simulink model "project3_v1_CoSim"  (R2021a)
settings: Solver=VariableStepAuto  StartTime=0.0  StopTime=30  RelTol=1e-3
undefined symbols (not defined in the file or in its folder): A, N
libraries: hdlBasic x25, xbsIndex_r4 x1, JTAGRuntimeCosim_r4 x1
settings Model: Creator=caval  LastModifiedBy=hl116

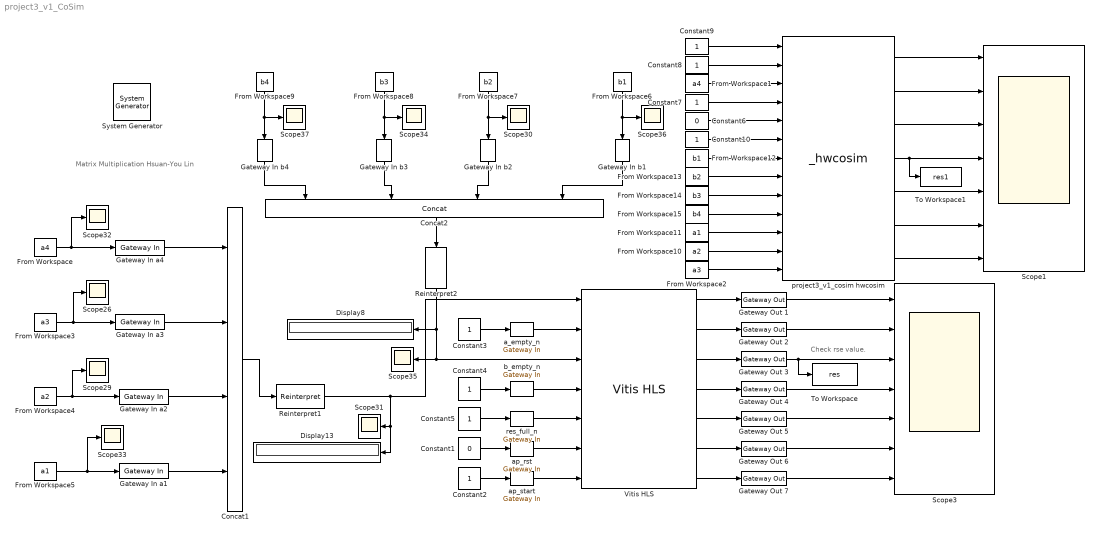
== system project3_v1_CoSim ==
  note: Matrix Multiplication
      | Hsuan-You Lin
  note: Check rse value.
  " System Generator" : xbsIndex_r4/ System Generator  Tag=genX  xilinxfamily=zynq  part=xc7z020  speed=-1  package=clg484  synthesis_tool=Vivado  clock_wrapper=Clock Enables  directory=./netlist_cosim  proj_type=Vivado  Synth_file=Vivado Synthesis Defaults  Impl_file=Vivado Implementation Defaults  testbench=off  simulink_period=1  sysclk_period=10  dcm_input_clock_period=10  incr_netlist=off  trim_vbits=Everywhere in SubSystem  dbl_ovrd=According to Block Masks  core_generation=According to Block Masks  run_coregen=off  deprecated_control=off  eval_field=0  block_type=sysgen
  Concat1 : hdlBasic/Concat  num_inputs=4  XmcBlockStatus=1  maskContainerNames=group1  block_type=concat  block_config=sysgen:Concat_config
  Concat2 : hdlBasic/Concat  num_inputs=4  XmcBlockStatus=1  maskContainerNames=group1  block_type=concat  block_config=sysgen:Concat_config
  Constant1 : Constant  Value=0
  Constant{2..5,7..10} (8 alike) : Constant
  Constant6 : Constant  Value=0
  Display13 : Display
      settings: Format=hex (Stored Integer)
  Display8 : Display
      settings: Format=hex (Stored Integer)
  From Workspace : FromWorkspace  VariableName=a4
  From Workspace1 : FromWorkspace  VariableName=a4
  From Workspace10 : FromWorkspace  VariableName=a2
  From Workspace11 : FromWorkspace  VariableName=a1
  From Workspace12 : FromWorkspace  VariableName=b1
  From Workspace13 : FromWorkspace  VariableName=b2
  From Workspace14 : FromWorkspace  VariableName=b3
  From Workspace15 : FromWorkspace  VariableName=b4
  From Workspace2 : FromWorkspace  VariableName=a3
  From Workspace3 : FromWorkspace  VariableName=a3
  From Workspace4 : FromWorkspace  VariableName=a2
  From Workspace5 : FromWorkspace  VariableName=a1
  From Workspace6 : FromWorkspace  VariableName=b1
  From Workspace7 : FromWorkspace  VariableName=b2
  From Workspace8 : FromWorkspace  VariableName=b3
  From Workspace9 : FromWorkspace  VariableName=b4
  Gateway In a{1..4} (4 alike) : hdlBasic/Gateway In  gui_display_data_type=Fixed-point  arith_type=Unsigned  n_bits=16  bin_pt=0  preci_type=Single  exp_width=8  frac_width=24  rows=1  columns=1  quantization="Round  (unbiased: +/- Inf)"  overflow=Saturate  period=1  UseAsADC=off  ADCChannel='1'  interface=None  automatic_assignment=on  address_offset=hex2dec('00')  intf_name=''  intf_description=''  default_value=0  timing_constraint=None  locs_specified=off  LOCs={}  io_standard={}  inherit_from_input=off  hdl_port=on  XmcBlockStatus=1  maskContainerNames=group4  block_type=gatewayin  block_config=sysgen:gateway_in_config  block_width_w=590  block_height_w=620  block_width=640  block_height=850
  Gateway In b{1..4} (4 alike) : hdlBasic/Gateway In  gui_display_data_type=Fixed-point  arith_type=Unsigned  n_bits=16  bin_pt=0  preci_type=Single  exp_width=8  frac_width=24  rows=1  columns=1  quantization="Round  (unbiased: +/- Inf)"  overflow=Saturate  period=1  UseAsADC=off  ADCChannel='1'  interface=None  automatic_assignment=on  address_offset=hex2dec('00')  intf_name=''  intf_description=''  default_value=0  timing_constraint=None  locs_specified=off  LOCs={}  io_standard={}  inherit_from_input=off  hdl_port=on  XmcBlockStatus=1  maskContainerNames=group4  block_type=gatewayin  block_config=sysgen:gateway_in_config  block_width_w=590  block_height_w=620  block_width=640  block_height=850
  Gateway Out {1..7} (7 alike) : hdlBasic/Gateway Out  inherit_from_input=on  hdl_port=on  rows=1  columns=1  UseAsDAC=off  DACChannel='1'  interface=None  automatic_assignment=on  address_offset=hex2dec('00')  intf_name=''  intf_description='Output_R'  timing_constraint=None  locs_specified=off  LOCs={}  io_standard={}  XmcBlockStatus=1  maskContainerNames=group4  block_type=gatewayout  block_config=sysgen:gateway_out_config  block_width_w=590  block_height_w=620  block_width=620  block_height=750
  Reinterpret1 : hdlBasic/Reinterpret  force_arith_type=on  arith_type="Signed  (2's comp)"  force_bin_pt=off  bin_pt=0  XmcBlockStatus=1  maskContainerNames=group1  block_type=reinterpret  block_config=sysgen:Reinterpret_config
  Reinterpret2 : hdlBasic/Reinterpret  force_arith_type=on  arith_type="Signed  (2's comp)"  force_bin_pt=off  bin_pt=0  XmcBlockStatus=1  maskContainerNames=group1  block_type=reinterpret  block_config=sysgen:Reinterpret_config
  Scope1 : Scope  NumInputPorts=7
  Scope{26,29..37} (10 alike) : Scope
  Scope3 : Scope  NumInputPorts=7
  To Workspace : ToWorkspace  VariableName=res  SaveFormat=Timeseries  SampleTime=-1
      settings: Save2DSignal=2-D array (concatenate along first dimension)
  To Workspace1 : ToWorkspace  VariableName=res1  SaveFormat=Timeseries  SampleTime=-1
      settings: Save2DSignal=2-D array (concatenate along first dimension)
  Vitis HLS : hdlBasic/Vitis HLS  anytable='.\Project3_v1_hls\solution4_Final'  fast_sim=off  display_datatype=off  rate_propagation_method=Simulink system period  model_file_path=''  latency=1  block_type=vitis_hls
      settings: infoedit=This block allows including C,C++ and SystemC source files in System Generator for DSP designs.
  "a_empty_n " : hdlBasic/Gateway In  gui_display_data_type=Boolean  arith_type=Boolean  n_bits=16  bin_pt=0  preci_type=Single  exp_width=8  frac_width=24  rows=1  columns=1  quantization="Round  (unbiased: +/- Inf)"  overflow=Saturate  period=1  UseAsADC=off  ADCChannel='1'  interface=None  automatic_assignment=on  address_offset=hex2dec('00')  intf_name=''  intf_description='Input_A'  default_value=0  timing_constraint=None  locs_specified=off  LOCs={}  io_standard={}  inherit_from_input=off  hdl_port=on  XmcBlockStatus=1  maskContainerNames=group4  block_type=gatewayin  block_config=sysgen:gateway_in_config  block_width_w=590  block_height_w=620  block_width=640  block_height=850
  ap_rst : hdlBasic/Gateway In  gui_display_data_type=Boolean  arith_type=Boolean  n_bits=16  bin_pt=0  preci_type=Single  exp_width=8  frac_width=24  rows=1  columns=1  quantization="Round  (unbiased: +/- Inf)"  overflow=Saturate  period=1  UseAsADC=off  ADCChannel='1'  interface=None  automatic_assignment=on  address_offset=hex2dec('00')  intf_name=''  intf_description='Input_A'  default_value=0  timing_constraint=None  locs_specified=off  LOCs={}  io_standard={}  inherit_from_input=off  hdl_port=on  XmcBlockStatus=1  maskContainerNames=group4  block_type=gatewayin  block_config=sysgen:gateway_in_config  block_width_w=590  block_height_w=620  block_width=640  block_height=850
  "ap_start " : hdlBasic/Gateway In  gui_display_data_type=Boolean  arith_type=Boolean  n_bits=16  bin_pt=0  preci_type=Single  exp_width=8  frac_width=24  rows=1  columns=1  quantization="Round  (unbiased: +/- Inf)"  overflow=Saturate  period=1  UseAsADC=off  ADCChannel='1'  interface=None  automatic_assignment=on  address_offset=hex2dec('00')  intf_name=''  intf_description='Input_A'  default_value=0  timing_constraint=None  locs_specified=off  LOCs={}  io_standard={}  inherit_from_input=off  hdl_port=on  XmcBlockStatus=1  maskContainerNames=group4  block_type=gatewayin  block_config=sysgen:gateway_in_config  block_width_w=590  block_height_w=620  block_width=640  block_height=850
  b_empty_n : hdlBasic/Gateway In  gui_display_data_type=Boolean  arith_type=Boolean  n_bits=16  bin_pt=0  preci_type=Single  exp_width=8  frac_width=24  rows=1  columns=1  quantization="Round  (unbiased: +/- Inf)"  overflow=Saturate  period=1  UseAsADC=off  ADCChannel='1'  interface=None  automatic_assignment=on  address_offset=hex2dec('00')  intf_name=''  intf_description='Input_A'  default_value=0  timing_constraint=None  locs_specified=off  LOCs={}  io_standard={}  inherit_from_input=off  hdl_port=on  XmcBlockStatus=1  maskContainerNames=group4  block_type=gatewayin  block_config=sysgen:gateway_in_config  block_width_w=590  block_height_w=620  block_width=640  block_height=850
  project3_v1_cosim hwcosim : JTAGRuntimeCosim_r4/_hwcosim  clkSrc=Single Stepped  hasCombinationalPath=on  bitfileName=C:\ELEC522\am251\proj3\netlist\project3_cosim.bit  skipConfig=off  dispPartInfo=off  useZynqReconfigScript=on  cable=Auto Detect  speed=N/A  cablePort=N/A  cableLocation=Local  shareCable=off  xmp=[]  software_settings=[]  design_xtable=|  binDir=[]  engineDll=JTAGCosimEngine.dll  cableWaitTime=10  bscanPos=-1  IRLengths=[]  useWaitBox=1  hasBufgmux=on  Scheme=Cosim  useCmdProc=1  hasProc=0  useImpact=0  printLogFile=0  userChain=2  XmcBlockStatus=0  maskContainerNames=tabcontainer1  block_type=jtagcosim  block_config=Sysgen:hwcosim_block_config
      | {
      |     'clkWrapper' => 'project3_cosim',
      |     'burstMode' => false,
      |     'burstFifoDepth' => '1024',
      |     'shared_memories' => {},
      |     'clocksGcd' => 1,
      |     'device' => {
      |       'family' => 'zynq',
      |       'part' => 'xc7z020',
      |       'package' => 'clg484',
      |       'speed' => '-1',
      |     },
      |     'ports' => {
      |       'aempty' => {
      |         'direction' => 'in',
      |         'width' => 1,
      |         'name' => 'aempty',
      |         'period' => 1,
      |         'icon_text' => 'aempty',
      |         'type' => 'Bool',
      |         'arithmetic_type' => 'xlUnsigned',
      |         'dat_file' => 'project3_cosim_aempty.dat',
      |         'bin_pt' => 0,
      |         'addr_offset' => 0,
      |         'bd_port_index' => 0,
      |       },
      |       'resfull' => {
      |         'direction' => 'in',
      |         'width' => 1,
      |         'name' => 'resfull',
      |         'period' => 1,
      |         'icon_text' => 'resfull',
      |         'type' => 'Bool',
      |         'arithmetic_type' => 'xlUnsigned',
      |         'dat_file' => 'project3_cosim_resfull.dat',
      |         'bin_pt' => 0,
      |         'addr_offset' => 4,
      |         'bd_port_index' => 1,
      |       },
      |       'input_a4' => {
      |         'direction' => 'in',
      |         'width' => 16,
      |         'name' => 'input_a4',
      |         'period' => 1,
      |         'icon_text' => 'Input_A4',
      |         'type' => 'UFix_16_0',
      |         'arithmetic_type' => 'xlUnsigned',
      |         'dat_file' => 'project3_cosim_input_a4.dat',
      |         'bin_pt' => 0,
      |         'addr_offset' => 8,
      |         'bd_port_index' => 2,
      |       },
      |       'start' => {
      |         'direction' => 'in',
      |         'width' => 1,
      |         'name' => 'start',
      |         'period' => 1,
      |         'icon_text' => 'start',
      |         'type' => 'Bool',
      |         'arithmetic_type' => 'xlUnsigned',
      |         'dat_file' => 'project3_cosim_start.dat',
      |         'bin_pt' => 0,
      |         'addr_offset' => 12,
      |         'bd_port_index' => 3,
      |       },
      |       'reset' => {
      |         'direction' => 'in',
      |         'width' => 1,
      |         'name' => 'reset',
      |         'period' => 1,
      |         'icon_text' => 'reset',
      |         'type' => 'Bool',
      |         'arithmetic_type' => 'xlUnsigned',
      |         'dat_file' => 'project3_cosim_reset.dat',
      |         'bin_pt' => 0,
      |         'addr_offset' => 16,
      |         'bd_port_index' => 4,
      |       },
      |       'bempty' => {
      |         'direction' => 'in',
      |         'width' => 1,
      |         'name' => 'bempty',
      |         'period' => 1,
      |         'icon_text' => 'bempty',
      |         'type' => 'Bool',
      |         'arithmetic_type' => 'xlUnsigned',
      |         'dat_file' => 'project3_cosim_bempty.dat',
      |         'bin_pt' => 0,
      |         'addr_offset' => 20,
      |         'bd_port_index' => 5,
      |       },
      |       'input_b1' => {
      |         'direction' => 'in',
      |         'width' => 16,
      |         'name' => 'input_b1',
      |         'period' => 1,
      |         'icon_text' => 'Input_B1',
      |         'type' => 'UFix_16_0',
      |         'arithmetic_type' => 'xlUnsigned',
      |         'dat_file' => 'project3_cosim_input_b1.dat',
      |         'bin_pt' => 0,
      |         'addr_offset' => 24,
      |         'bd_port_index' => 6,
      |       },
      |       'input_b2' => {
      |         'direction' => 'in',
      |         'width' => 16,
      |         'name' => 'input_b2',
      |         'period' => 1,
      |         'icon_text' => 'Input_B2',
      |         'type' => 'UFix_16_0',
      |         'arithmetic_type' => 'xlUnsigned',
      |         'dat_file' => 'project3_cosim_input_b2.dat',
      |         'bin_pt' => 0,
      |         'addr_offset' => 28,
      |         'bd_port_index' => 7,
      |       },
      |       'input_b3' => {
      |         'direction' => 'in',
      |         'width' => 16,
      |         'name' => 'input_b3',
      |         'period' => 1,
      |         'icon_text' => 'Input_B3',
      |         'type' => 'UFix_16_0',
      |         'arithmetic_type' => 'xlUnsigned',
      |         'dat_file' => 'project3_cosim_input_b3.dat',
      |         'bin_pt' => 0,
      |         'addr_offset' => 32,
      |         'bd_port_index' => 8,
      |       },
      |       'input_b4' => {
      |         'direction' => 'in',
      |         'width' => 16,
      |         'name' => 'input_b4',
      |         'period' => 1,
      |         'icon_text' => 'Input_B4',
      |         'type' => 'UFix_16_0',
      |         'arithmetic_type' => 'xlUnsigned',
      |         'dat_file' => 'project3_cosim_input_b4.dat',
      |         'bin_pt' => 0,
      |         'addr_offset' => 36,
      |         'bd_port_index' => 9,
      |       },
      |       'input_a1' => {
      |         'direction' => 'in',
      |         'width' => 16,
      |         'name' => 'input_a1',
      |         'period' => 1,
      |         'icon_text' => 'Input_A1',
      |         'type' => 'UFix_16_0',
      |         'arithmetic_type' => 'xlUnsigned',
      |         'dat_file' => 'project3_cosim_input_a1.dat',
      |         'bin_pt' => 0,
      |         'addr_offset' => 40,
      |         'bd_port_index' => 10,
      |       },
      |       'input_a2' => {
      |         'direction' => 'in',
      |         'width' => 16,
      |         'name' => 'input_a2',
      |         'period' => 1,
      |         'icon_text' => 'Input_A2',
      |         'type' => 'UFix_16_0',
      |         'arithmetic_type' => 'xlUnsigned',
      |         'dat_file' => 'project3_cosim_input_a2.dat',
      |         'bin_pt' => 0,
      |         'addr_offset' => 44,
      |         'bd_port_index' => 11,
      |       },
      |       'input_a3' => {
      |         'direction' => 'in',
      |         'width' => 16,
      |         'name' => 'input_a3',
      |         'period' => 1,
      |         'icon_text' => 'Input_A3',
      |         'type' => 'UFix_16_0',
      |         'arithmetic_type' => 'xlUnsigned',
      |         'dat_file' => 'project3_cosim_input_a3.dat',
      |         'bin_pt' => 0,
      |         'addr_offset' => 48,
      |         'bd_port_index' => 12,
      |       },
      |       'idle' => {
      |         'direction' => 'out',
      |         'width' => 1,
      |         'name' => 'idle',
      |         'period' => 1,
      |         'icon_text' => 'idle',
      |         'type' => 'Bool',
      |         'arithmetic_type' => 'xlUnsigned',
      |         'dat_file' => 'project3_cosim_idle.dat',
      |         'bin_pt' => 0,
      |         'addr_offset' => 52,
      |         'bd_port_index' => 0,
      |       },
      |       'bread' => {
      |         'direction' => 'out',
      |         'width' => 1,
      |         'name' => 'bread',
      |         'period' => 1,
      |         'icon_text' => 'bread',
      |         'type' => 'Bool',
      |         'arithmetic_type' => 'xlUnsigned',
      |         'dat_file' => 'project3_cosim_bread.dat',
      |         'bin_pt' => 0,
      |         'addr_offset' => 56,
      |         'bd_port_index' => 1,
      |       },
      |       'ready' => {
      |         'direction' => 'out',
      |         'width' => 1,
      |         'name' => 'ready',
      |         'period' => 1,
      |         'icon_text' => 'ready',
      |         'type' => 'Bool',
      |         'arithmetic_type' => 'xlUnsigned',
      |         'dat_file' => 'project3_cosim_ready.dat',
      |         'bin_pt' => 0,
      |         'addr_offset' => 60,
      |         'bd_port_index' => 2,
      |       },
      |       'res' => {
      |         'direction' => 'out',
      |         'width' => 64,
      |         'name' => 'res',
      |         'period' => 1,
      |         'icon_text' => 'res',
      |         'type' => 'Fix_64_0',
      |         'arithmetic_type' => 'xlSigned',
      |         'dat_file' => 'project3_cosim_res.dat',
      |         'bin_pt' => 0,
      |         'addr_offset' => 64,
      |         'bd_port_index' => 3,
      |       },
      |       'reswrite' => {
      |         'direction' => 'out',
      |         'width' => 1,
      |         'name' => 'reswrite',
      |         'period' => 1,
      |         'icon_text' => 'reswrite',
      |         'type' => 'Bool',
      |         'arithmetic_type' => 'xlUnsigned',
      |         'dat_file' => 'project3_cosim_reswrite.dat',
      |         'bin_pt' => 0,
      |         'addr_offset' => 72,
      |         'bd_port_index' => 4,
      |       },
      |       'done' => {
      |         'direction' => 'out',
      |         'width' => 1,
      |         'name' => 'done',
      |         'period' => 1,
      |         'icon_text' => 'done',
      |         'type' => 'Bool',
      |         'arithmetic_type' => 'xlUnsigned',
      |         'dat_file' => 'project3_cosim_done.dat',
      |         'bin_pt' => 0,
      |         'addr_offset' => 76,
      |         'bd_port_index' => 5,
      |       },
      |       'aread' => {
      |         'direction' => 'out',
      |         'width' => 1,
      |         'name' => 'aread',
      |         'period' => 1,
      |         'icon_text' => 'aread',
      |         'type' => 'Bool',
      |         'arithmetic_type' => 'xlUnsigned',
      |         'dat_file' => 'project3_cosim_aread.dat',
      |         'bin_pt' => 0,
      |         'addr_offset' => 80,
      |         'bd_port_index' => 6,
      |       },
      |     },
      |   }
  res_full_n : hdlBasic/Gateway In  gui_display_data_type=Boolean  arith_type=Boolean  n_bits=16  bin_pt=0  preci_type=Single  exp_width=8  frac_width=24  rows=1  columns=1  quantization="Round  (unbiased: +/- Inf)"  overflow=Saturate  period=1  UseAsADC=off  ADCChannel='1'  interface=None  automatic_assignment=on  address_offset=hex2dec('00')  intf_name=''  intf_description='Input_A'  default_value=0  timing_constraint=None  locs_specified=off  LOCs={}  io_standard={}  inherit_from_input=off  hdl_port=on  XmcBlockStatus=1  maskContainerNames=group4  block_type=gatewayin  block_config=sysgen:gateway_in_config  block_width_w=590  block_height_w=620  block_width=640  block_height=850
  wires:
  Constant1/1 -> ap_rst/1
  Constant2/1 -> "ap_start "/1
  From Workspace4/1 -> Scope29/1, Gateway In a2/1
  From Workspace5/1 -> Scope33/1, Gateway In a1/1
  Gateway In a4/1 -> Concat1/1
  Gateway In a3/1 -> Concat1/2
  Gateway In a2/1 -> Concat1/3
  Gateway In a1/1 -> Concat1/4
  From Workspace3/1 -> Scope26/1, Gateway In a3/1
  Reinterpret1/1 -> Display13/1, Scope31/1, Vitis HLS/1
  Concat1/1 -> Reinterpret1/1
  From Workspace/1 -> Gateway In a4/1, Scope32/1
  From Workspace8/1 -> Gateway In b3/1, Scope34/1
  From Workspace7/1 -> Scope30/1, Gateway In b2/1
  Concat2/1 -> Reinterpret2/1
  From Workspace6/1 -> Gateway In b1/1, Scope36/1
  From Workspace9/1 -> Scope37/1, Gateway In b4/1
  Gateway In b4/1 -> Concat2/1
  Gateway In b3/1 -> Concat2/2
  Gateway In b2/1 -> Concat2/3
  Gateway In b1/1 -> Concat2/4
  Constant3/1 -> "a_empty_n "/1
  Constant4/1 -> b_empty_n/1
  Constant5/1 -> res_full_n/1
  Vitis HLS/2 -> Gateway Out 2/1
  Vitis HLS/1 -> Gateway Out 1/1
  Vitis HLS/3 -> Gateway Out 3/1
  Vitis HLS/4 -> Gateway Out 4/1
  Vitis HLS/5 -> Gateway Out 5/1
  Vitis HLS/7 -> Gateway Out 7/1
  Gateway Out 3/1 -> To Workspace/1, Scope3/3
  Gateway Out 2/1 -> Scope3/2
  Gateway Out 1/1 -> Scope3/1
  Gateway Out 4/1 -> Scope3/4
  Gateway Out 5/1 -> Scope3/5
  Gateway Out 7/1 -> Scope3/7
  Vitis HLS/6 -> Gateway Out 6/1
  Gateway Out 6/1 -> Scope3/6
  "a_empty_n "/1 -> Vitis HLS/2
  b_empty_n/1 -> Vitis HLS/4
  res_full_n/1 -> Vitis HLS/5
  ap_rst/1 -> Vitis HLS/6
  "ap_start "/1 -> Vitis HLS/7
  Reinterpret2/1 -> Display8/1, Scope35/1, Vitis HLS/3
  From Workspace10/1 -> project3_v1_cosim hwcosim/12
  From Workspace2/1 -> project3_v1_cosim hwcosim/13
  From Workspace11/1 -> project3_v1_cosim hwcosim/11
  From Workspace1/1 -> project3_v1_cosim hwcosim/3
  From Workspace12/1 -> project3_v1_cosim hwcosim/7
  From Workspace13/1 -> project3_v1_cosim hwcosim/8
  From Workspace14/1 -> project3_v1_cosim hwcosim/9
  From Workspace15/1 -> project3_v1_cosim hwcosim/10
  Constant6/1 -> project3_v1_cosim hwcosim/5
  Constant7/1 -> project3_v1_cosim hwcosim/4
  Constant8/1 -> project3_v1_cosim hwcosim/2
  Constant9/1 -> project3_v1_cosim hwcosim/1
  Constant10/1 -> project3_v1_cosim hwcosim/6
  project3_v1_cosim hwcosim/4 -> Scope1/4, To Workspace1/1
  project3_v1_cosim hwcosim/7 -> Scope1/7
  project3_v1_cosim hwcosim/6 -> Scope1/6
  project3_v1_cosim hwcosim/5 -> Scope1/5
  project3_v1_cosim hwcosim/3 -> Scope1/3
  project3_v1_cosim hwcosim/2 -> Scope1/2
  project3_v1_cosim hwcosim/1 -> Scope1/1
